simulink model "actuatorController"  (R2025b)
settings: Solver=FixedStepDiscrete  StartTime=0.0  StopTime=3  FixedStep=1e-3  RelTol=1e-3
undefined symbols (not defined in the file or in its folder): controller_mode, controller_modes, controllerGains, DiscIntNeverNeededParam
libraries: simulink x10, metux_library x4, eeGeneralControl x3, simulink_extras x2
settings Model: Creator=karadeli  LastModifiedBy=karadeli
settings OptimizationCC: GainParamInheritBuiltInType=on  UseFloatMulNetSlope=on  DefaultUnderspecifiedDataType=single  PassReuseOutputArgsAs=Individual arguments  ZeroExternalMemoryAtStartup=off  ZeroInternalMemoryAtStartup=off  NoFixptDivByZeroProtection=on  EfficientFloat2IntCast=on  LifeSpan=1  OptimizeBlockOrder=speed  DifferentSizesBufferReuse=on  EfficientTunableParamExpr=on
settings DebuggingCC: ParamSuppressDoubleToSinglePrecisionLossMsg=on  ParameterTunabilityLossMsg=none
settings HardwareCC: ProdBitPerPointer=32.0  ProdBitPerSizeT=32.0  ProdBitPerPtrDiffT=32.0  ProdLargestAtomicInteger=Long  ProdLargestAtomicFloat=Double  ProdWordSize=32.0  ProdLongLongMode=on  ProdHWDeviceType=ARM Compatible->ARM Cortex-M
settings SFSimCC: MATLABDynamicMemAlloc=off
settings RTWCC: SystemTargetFile=ert.tlc  GenCodeOnly=on  TemplateMakefile=ert_default_tmf  TargetLang=C++  Description=Embedded Coder
settings CodeAppCC: ForceParamTrailComments=on  IgnoreCustomStorageClasses=off  OperatorAnnotations=on  SimulinkDataObjDesc=on  SFDataObjDesc=on  CustomSymbolStrGlobalVar=rt$N$M  CustomSymbolStrType=$N$M  CustomSymbolStrFcn=$N$M$F  CustomSymbolStrMacro=$N$M  InsertBlockDesc=on
settings ERTTargetCC: InlinedParameterPlacement=Hierarchical  RootIOFormat=Structure reference  ERTCustomFileTemplate=example_file_process.tlc  ERTFilePackagingFormat=CompactWithDataFile  TargetLangStandard=C++11 (ISO)  GenerateSampleERTMain=on  IncludeMdlTerminateFcn=off  CombineSignalStateStructs=on  SupportAbsoluteTime=off  CodeInterfacePackaging=C++ class  SubcomponentCodeInterfacePackaging=C++ class  SupportNonFinite=off  SupportComplex=off  SupportNonInlinedSFcns=on

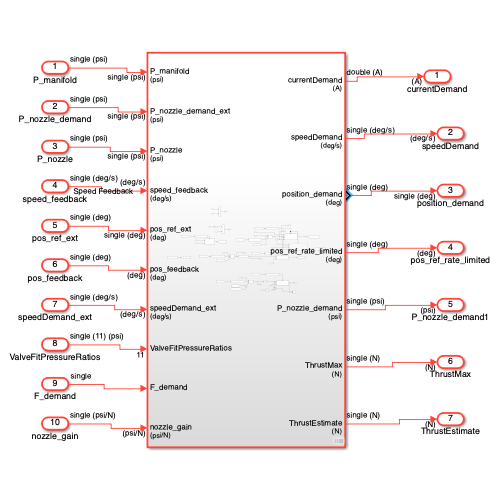
[thumbnail: Simulink's stored preview of the top-level diagram]
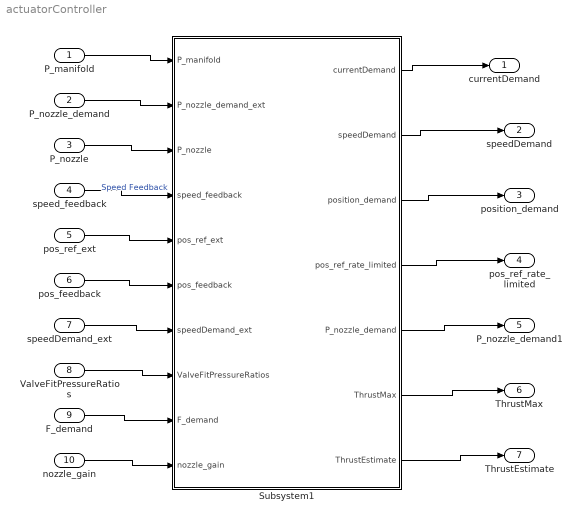
== system actuatorController ==
  P_manifold : Inport  OutDataTypeStr=single  Unit=psi  PortDimensions=1
  P_nozzle_demand : Inport  Port=2  OutDataTypeStr=single  Unit=psi  PortDimensions=1
  P_nozzle : Inport  Port=3  OutDataTypeStr=single  Unit=psi  PortDimensions=1
  speed_feedback : Inport  Port=4  Unit=deg/s  SampleTime=controllerGains.speed.Ts  Interpolate=off
  pos_ref_ext : Inport  Port=5  OutDataTypeStr=single  Unit=deg  SampleTime=controllerGains.position.Ts  Interpolate=off
  pos_feedback : Inport  Port=6  Unit=deg  SampleTime=controllerGains.position.Ts  Interpolate=off
  speedDemand_ext : Inport  Port=7  Unit=deg/s
  ValveFitPressureRatios : Inport  Port=8
  F_demand : Inport  Port=9
  nozzle_gain : Inport  Port=10  Unit=psi/N
  Subsystem1 : Subsystem
  currentDemand : Outport  Unit=A
  speedDemand : Outport  Port=2  Unit=deg/s
  position_demand : Outport  Port=3  OutDataTypeStr=single  Unit=deg
  pos_ref_rate_limited : Outport  Port=4  Unit=deg
  P_nozzle_demand1 : Outport  Port=5  Unit=psi
  ThrustMax : Outport  Port=6  Unit=N
  ThrustEstimate : Outport  Port=7  Unit=N
  wires:
  speed_feedback/1 -> Subsystem1/4(speed_feedback)  "Speed Feedback"
  pos_ref_ext/1 -> Subsystem1/5(pos_ref_ext)
  pos_feedback/1 -> Subsystem1/6(pos_feedback)
  P_manifold/1 -> Subsystem1/1(P_manifold)
  P_nozzle_demand/1 -> Subsystem1/2(P_nozzle_demand_ext)
  P_nozzle/1 -> Subsystem1/3(P_nozzle)
  speedDemand_ext/1 -> Subsystem1/7(speedDemand_ext)
  Subsystem1/3(position_demand) -> position_demand/1
  Subsystem1/4(pos_ref_rate_limited) -> pos_ref_rate_limited/1
  Subsystem1/1(currentDemand) -> currentDemand/1
  Subsystem1/2(speedDemand) -> speedDemand/1
  ValveFitPressureRatios/1 -> Subsystem1/8(ValveFitPressureRatios)
  F_demand/1 -> Subsystem1/9(F_demand)
  nozzle_gain/1 -> Subsystem1/10(nozzle_gain)
  Subsystem1/5(P_nozzle_demand) -> P_nozzle_demand1/1
  Subsystem1/6(ThrustMax) -> ThrustMax/1
  Subsystem1/7(ThrustEstimate) -> ThrustEstimate/1

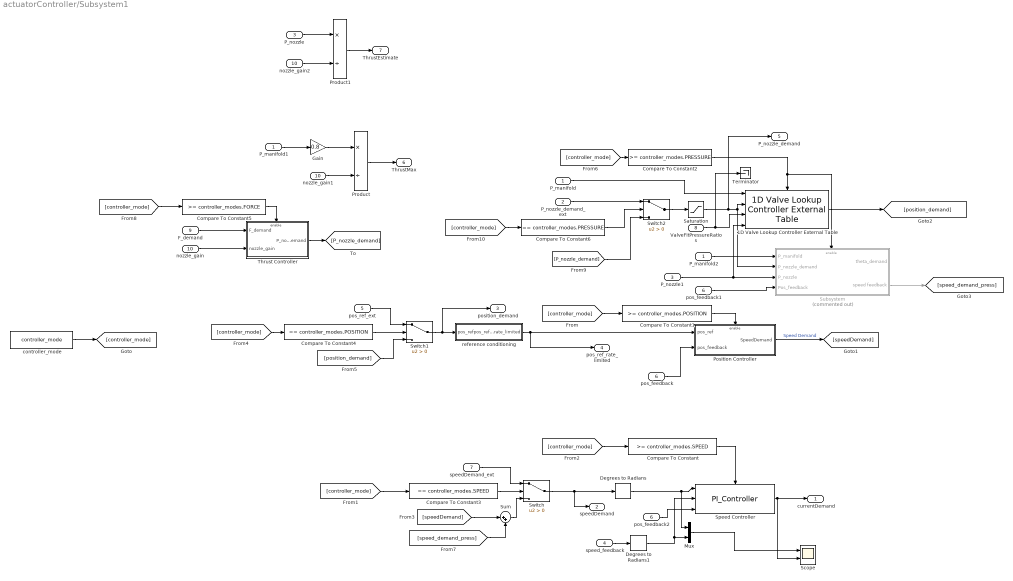
== system actuatorController/Subsystem1 ==
  P_manifold : Inport  OutDataTypeStr=single  Unit=psi  PortDimensions=1
  P_nozzle_demand_ext : Inport  Port=2  OutDataTypeStr=single  Unit=psi  PortDimensions=1
  P_nozzle : Inport  Port=3  OutDataTypeStr=single  Unit=psi  PortDimensions=1
  speed_feedback : Inport  Port=4  Unit=deg/s  SampleTime=controllerGains.speed.Ts  Interpolate=off
  pos_ref_ext : Inport  Port=5  OutDataTypeStr=single  Unit=deg  SampleTime=controllerGains.position.Ts  Interpolate=off
  pos_feedback : Inport  Port=6  Unit=deg  SampleTime=controllerGains.position.Ts  Interpolate=off
  speedDemand_ext : Inport  Port=7  Unit=deg/s
  ValveFitPressureRatios : Inport  Port=8
  F_demand : Inport  Port=9
  nozzle_gain : Inport  Port=10  Unit=psi/N
  1D Valve Lookup Controller External Table : metux_library/1D Valve Lookup Controller External Table  SystemSampleTime=-1  VariantActivationTime=update diagram  EmptyChoice=off  PassThrough=off  PassThroughVariantControl=(default)  EmptyChoiceVariantControl=(default)  AllowFlexibleInterface=on  Latency=0  AutoFrameSizeCalculation=off
  Compare To Constant : simulink/Logic and Bit Operations/Compare To Constant  relop=>=  const=controller_modes.SPEED  OutDataTypeStr=boolean
  Compare To Constant1 : simulink/Logic and Bit Operations/Compare To Constant  relop=>=  const=controller_modes.POSITION  OutDataTypeStr=boolean
  Compare To Constant2 : simulink/Logic and Bit Operations/Compare To Constant  relop=>=  const=controller_modes.PRESSURE  OutDataTypeStr=boolean
  Compare To Constant3 : simulink/Logic and Bit Operations/Compare To Constant  relop===  const=controller_modes.SPEED  OutDataTypeStr=boolean
  Compare To Constant4 : simulink/Logic and Bit Operations/Compare To Constant  relop===  const=controller_modes.POSITION  OutDataTypeStr=boolean
  Compare To Constant5 : simulink/Logic and Bit Operations/Compare To Constant  relop=>=  const=controller_modes.FORCE  OutDataTypeStr=boolean
  Compare To Constant6 : simulink/Logic and Bit Operations/Compare To Constant  relop===  const=controller_modes.PRESSURE  OutDataTypeStr=boolean
  Degrees to Radians : simulink_extras/Transformations/Degrees to Radians
  Degrees to Radians1 : simulink_extras/Transformations/Degrees to Radians
  Gain : Gain  Gain=0.8
  Mux : Mux  Inputs=2
  P_manifold1 : InportShadow  OutDataTypeStr=single  Unit=psi  PortDimensions=1
  P_manifold2 : InportShadow  OutDataTypeStr=single  Unit=psi  PortDimensions=1
  P_nozzle1 : InportShadow  Port=3  OutDataTypeStr=single  Unit=psi  PortDimensions=1
  Position Controller : Subsystem
  Product : Product  Inputs=*/
  Product1 : Product  Inputs=*/
  Saturation : Saturate  UpperLimit=1800  LowerLimit=0
  Scope : Scope  NumInputPorts=2
      settings: ActiveDisplayYMinimum=-3482.2818450927725  ActiveDisplayYMaximum=28164.697982788086
  Speed Controller : metux_library/PI_Controller  Kp=controllerGains.speed.Kp  Ki=controllerGains.speed.Ki  SatMax=controllerGains.speed.SatMax  SatMin=controllerGains.speed.SatMin  Ts=controllerGains.speed.Ts  RateLimiterMax=controllerGains.speed.RateLimiterMax  RateLimiterMin=controllerGains.speed.RateLimiterMin
  Subsystem : Subsystem  Commented=on
  Sum : Sum  Inputs=|++
  Switch : Switch  Criteria=u2 > Threshold  SaturateOnIntegerOverflow=off  InputSameDT=off
  Switch1 : Switch  Criteria=u2 > Threshold  SaturateOnIntegerOverflow=off  InputSameDT=off
  Switch2 : Switch  Criteria=u2 > Threshold  SaturateOnIntegerOverflow=off  InputSameDT=off
  Terminator : Terminator
  Thrust Controller : Subsystem
  controller_mode : Constant  Value=controller_mode  SampleTime=-1
  nozzle_gain1 : InportShadow  Port=10  Unit=psi/N
  nozzle_gain2 : InportShadow  Port=10  Unit=psi/N
  pos_feedback1 : InportShadow  Port=6  Unit=deg  SampleTime=controllerGains.position.Ts  Interpolate=off
  pos_feedback2 : InportShadow  Port=6  Unit=deg  SampleTime=controllerGains.position.Ts  Interpolate=off
  reference conditioning : Subsystem
  currentDemand : Outport  Unit=A
  speedDemand : Outport  Port=2  Unit=deg/s
  position_demand : Outport  Port=3  OutDataTypeStr=single  Unit=deg
  pos_ref_rate_limited : Outport  Port=4  Unit=deg
  P_nozzle_demand : Outport  Port=5  Unit=psi
  ThrustMax : Outport  Port=6  Unit=N
  ThrustEstimate : Outport  Port=7  Unit=N
  wires:
  P_nozzle_demand_ext/1 -> Switch2/1
  [controller_mode] -> Compare To Constant4/1
  controller_mode/1 -> [controller_mode]
  speedDemand_ext/1 -> Switch/1
  Mux/1 -> Scope/1
  Sum/1 -> Switch/3
  speed_feedback/1 -> Degrees to Radians1/1
  Position Controller/1(SpeedDemand) -> [speedDemand]  "Speed Demand"
  Degrees to Radians/1 -> Mux/1, Speed Controller/1
  Switch/1 -> speedDemand/1, Degrees to Radians/1
  Compare To Constant1/1 -> Position Controller/Enable
  [controller_mode] -> Compare To Constant2/1
  Compare To Constant/1 -> Speed Controller/Enable
  pos_feedback/1 -> Position Controller/2(pos_feedback)
  Compare To Constant2/1 -> Subsystem/Enable, 1D Valve Lookup Controller External Table/Enable
  Compare To Constant4/1 -> Switch1/2
  [position_demand] -> Switch1/3
  [controller_mode] -> Compare To Constant1/1
  Speed Controller/1 -> currentDemand/1, Scope/2
  [controller_mode] -> Compare To Constant/1
  pos_ref_ext/1 -> Switch1/1
  Switch1/1 -> position_demand/1, reference conditioning/1(pos_ref)
  Degrees to Radians1/1 -> Speed Controller/2, Mux/2
  [controller_mode] -> Compare To Constant3/1
  Compare To Constant3/1 -> Switch/2
  reference conditioning/1(pos_ref_rate_limited) -> pos_ref_rate_limited/1, Position Controller/1(pos_ref)
  [speedDemand] -> Sum/1
  [speed_demand_press] -> Sum/2
  P_manifold/1 -> 1D Valve Lookup Controller External Table/1
  [controller_mode] -> Compare To Constant5/1
  Compare To Constant5/1 -> Thrust Controller/Enable
  ValveFitPressureRatios/1 -> Terminator/1, 1D Valve Lookup Controller External Table/3
  F_demand/1 -> Thrust Controller/1(F_demand)
  nozzle_gain/1 -> Thrust Controller/2(nozzle_gain)
  Thrust Controller/1(P_nozzle_demand) -> [P_nozzle_demand]
  Switch2/1 -> Saturation/1
  Compare To Constant6/1 -> Switch2/2
  [controller_mode] -> Compare To Constant6/1
  [P_nozzle_demand] -> Switch2/3
  P_manifold1/1 -> Gain/1
  nozzle_gain1/1 -> Product/2
  Product/1 -> ThrustMax/1
  Gain/1 -> Product/1
  P_nozzle/1 -> Product1/1
  nozzle_gain2/1 -> Product1/2
  Product1/1 -> ThrustEstimate/1
  P_nozzle1/1 -> 1D Valve Lookup Controller External Table/4, Subsystem/3(P_nozzle)
  pos_feedback1/1 -> Subsystem/4(Pos_feedback)
  P_manifold2/1 -> Subsystem/1(P_manifold)
  Subsystem/2(speed feedback) -> [speed_demand_press]
  1D Valve Lookup Controller External Table/1 -> [position_demand]
  pos_feedback2/1 -> Speed Controller/3
  Saturation/1 -> P_nozzle_demand/1, Subsystem/2(P_nozzle_demand), 1D Valve Lookup Controller External Table/2

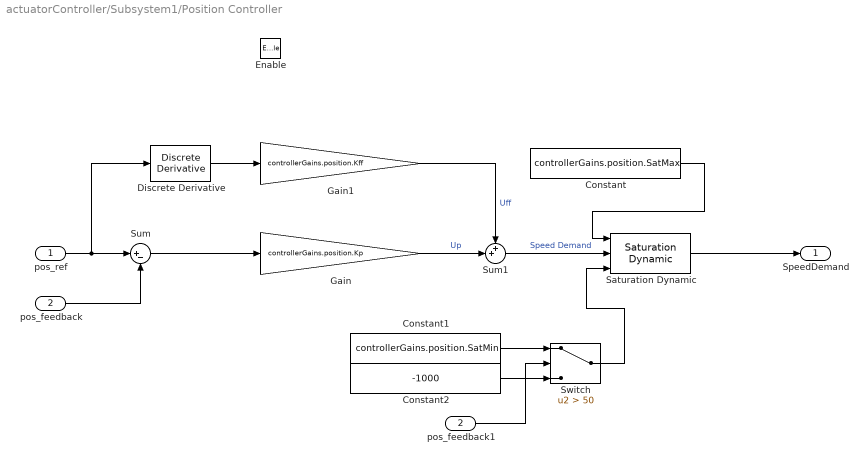
== system actuatorController/Subsystem1/Position Controller ==
  pos_ref : Inport  Unit=deg
  pos_feedback : Inport  Port=2  Unit=deg
  Enable : EnablePort  StatesWhenEnabling=reset
  Constant : Constant  Value=controllerGains.position.SatMax
  Constant1 : Constant  Value=controllerGains.position.SatMin
  Constant2 : Constant  Value=-1000  OutDataTypeStr=single
  Discrete Derivative : simulink/Discrete/Discrete Derivative  gainval=1.0  ICPrevScaledInput=0.0  OutMin=[]  OutMax=[]  OutDataType=fixdt(1, 16)  OutScaling=2^-10  DoSatur=off
  Gain : Gain  Gain=controllerGains.position.Kp
  Gain1 : Gain  Gain=controllerGains.position.Kff
  Saturation Dynamic : simulink/Discontinuities/Saturation Dynamic  OutMin=[]  OutMax=[]  OutDataTypeStr=Inherit: Same as second input  OutDataType=fixdt(1, 16)  OutScaling=2^-10  DoSatur=off
  Sum : Sum  Inputs=|+-
  Sum1 : Sum  Inputs=++|
  Switch : Switch  Criteria=u2 > Threshold  Threshold=50  SaturateOnIntegerOverflow=off  InputSameDT=off
  pos_feedback1 : InportShadow  Port=2  Unit=deg
  SpeedDemand : Outport  Unit=deg/s  OutputWhenDisabled=reset  InitialOutput=[0.0]
  wires:
  Saturation Dynamic/1 -> SpeedDemand/1
  pos_feedback/1 -> Sum/2
  Gain/1 -> Sum1/2  "Up"
  Sum/1 -> Gain/1
  pos_ref/1 -> Discrete Derivative/1, Sum/1
  Sum1/1 -> Saturation Dynamic/2  "Speed Demand"
  Discrete Derivative/1 -> Gain1/1
  Gain1/1 -> Sum1/1  "Uff"
  Constant/1 -> Saturation Dynamic/1
  Switch/1 -> Saturation Dynamic/3
  Constant1/1 -> Switch/1
  Constant2/1 -> Switch/3
  pos_feedback1/1 -> Switch/2

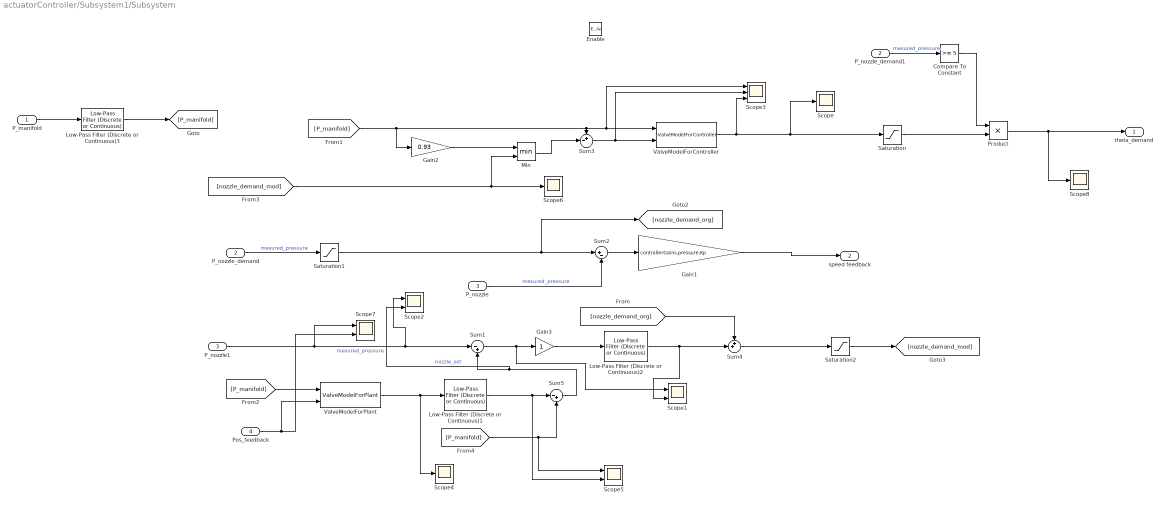
== system actuatorController/Subsystem1/Subsystem ==
  P_manifold : Inport
  P_nozzle_demand : Inport  Port=2
  P_nozzle : Inport  Port=3
  Pos_feedback : Inport  Port=4
  Enable : EnablePort  StatesWhenEnabling=reset
  Compare To Constant : simulink/Logic and Bit Operations/Compare To Constant  relop=>=  const=5  OutDataTypeStr=boolean
  Gain1 : Gain  Gain=controllerGains.pressure.Kp
  Gain2 : Gain  Gain=0.93
  Gain3 : Gain
  Low-Pass Filter (Discrete or Continuous)1 : eeGeneralControl/Low-Pass Filter (Discrete or Continuous)  K=1  T=0.001  B=inf  A=-inf  init_option=Inherited from block input  x0=0  Ts=-1
  Low-Pass Filter (Discrete or Continuous)2 : eeGeneralControl/Low-Pass Filter (Discrete or Continuous)  K=1  T=0.004  B=250  A=-250  init_option=Inherited from block input  x0=0  Ts=-1
  Low-Pass Filter (Discrete or Continuous)3 : eeGeneralControl/Low-Pass Filter (Discrete or Continuous)  K=single(1)  T=single(0.005)  B=inf  A=-inf  init_option=Inherited from block input  x0=0  Ts=-1
  Min : MinMax  Inputs=2
  P_nozzle1 : InportShadow  Port=3
  P_nozzle_demand1 : InportShadow  Port=2
  Product : Product
  Saturation : Saturate  UpperLimit=1080  LowerLimit=0
  Saturation1 : Saturate  UpperLimit=4000  LowerLimit=0
  Saturation2 : Saturate  UpperLimit=4000  LowerLimit=0
  Scope{,4,6,8} (4 alike) : Scope
      Scope settings: ActiveDisplayYMinimum=-15.395192146301266  ActiveDisplayYMaximum=138.55672931671143  DataLoggingVariableName=ScopeData2
      Scope4 settings: ActiveDisplayYMinimum=1007.1971893310547  ActiveDisplayYMaximum=2357.6605987548828  DataLoggingVariableName=ScopeData6
      Scope6 settings: ActiveDisplayYMinimum=-112.49999999999997  ActiveDisplayYMaximum=1012.5  DataLoggingVariableName=ScopeData8
      Scope8 settings: ActiveDisplayYMinimum=-18.167575836181637  ActiveDisplayYMaximum=163.50818252563477  DataLoggingVariableName=ScopeData10
  Scope{1..2,5,7} (4 alike) : Scope  NumInputPorts=2
      Scope1 settings: ActiveDisplayYMinimum=16.466037750244148  ActiveDisplayYMaximum=359.39812850952148  DataLoggingVariableName=ScopeData4
      Scope2 settings: ActiveDisplayYMinimum=-179.26073789596555  ActiveDisplayYMaximum=1025.8466792106628  DataLoggingVariableName=ScopeData5
      Scope5 settings: ActiveDisplayYMinimum=1218.2213745117188  ActiveDisplayYMaximum=2587.3870239257812  DataLoggingVariableName=ScopeData7
      Scope7 settings: ActiveDisplayYMinimum=-62.757351875305176  ActiveDisplayYMaximum=64.080883979797363  DataLoggingVariableName=ScopeData9
  Scope3 : Scope  NumInputPorts=3
      settings: ActiveDisplayYMinimum=-431.94372558593739  ActiveDisplayYMaximum=3887.4935302734375  DataLoggingVariableName=ScopeData3
  Sum1 : Sum  Inputs=|-+
  Sum2 : Sum  Inputs=|+-
  Sum3 : Sum  Inputs=+-|  OutDataTypeStr=single
  Sum4 : Sum  Inputs=++|
  Sum5 : Sum  Inputs=|-+
  ValveModelForController : metux_library/ValveModelForController  alpha=51.8534  C_max=0.9197
  ValveModelForPlant : metux_library/ValveModelForPlant  C_max=0.9197  alpha=51.8534
  theta_demand : Outport  OutputWhenDisabled=reset  InitialOutput=0
  speed feedback : Outport  Port=2
  wires:
  Sum1/1 -> Gain3/1, Scope1/1
  Sum3/1 -> Scope3/2, ValveModelForController/2
  Low-Pass Filter (Discrete or Continuous)1/1 -> Sum5/1, Scope5/2
  ValveModelForPlant/1 -> Low-Pass Filter (Discrete or Continuous)1/1, Scope4/1
  P_nozzle/1 -> Sum2/2  "mesured_pressure"
  P_nozzle_demand1/1 -> Compare To Constant/1  "mesured_pressure"
  P_manifold/1 -> Low-Pass Filter (Discrete or Continuous)3/1
  [P_manifold] -> Sum3/1, Scope3/1, ValveModelForController/1, Gain2/1
  Saturation/1 -> Product/2
  Compare To Constant/1 -> Product/1
  Pos_feedback/1 -> ValveModelForPlant/2, Scope7/2
  [P_manifold] -> ValveModelForPlant/1
  Gain3/1 -> Low-Pass Filter (Discrete or Continuous)2/1
  Saturation2/1 -> [nozzle_demand_mod]
  Min/1 -> Sum3/2
  Low-Pass Filter (Discrete or Continuous)3/1 -> [P_manifold]
  Low-Pass Filter (Discrete or Continuous)2/1 -> Sum4/2, Scope1/2
  P_nozzle1/1 -> Sum1/1, Scope2/1, Scope7/1  "mesured_pressure"
  Gain2/1 -> Min/1
  [nozzle_demand_mod] -> Scope6/1, Min/2
  Sum5/1 -> Sum1/2, Scope2/2  "nozzle_est"
  Saturation1/1 -> [nozzle_demand_org], Sum2/1
  [P_manifold] -> Sum5/2, Scope5/1
  ValveModelForController/1 -> Scope3/3, Saturation/1, Scope/1
  Product/1 -> theta_demand/1, Scope8/1
  Sum2/1 -> Gain1/1
  [nozzle_demand_org] -> Sum4/1
  P_nozzle_demand/1 -> Saturation1/1  "mesured_pressure"
  Sum4/1 -> Saturation2/1
  Gain1/1 -> speed feedback/1

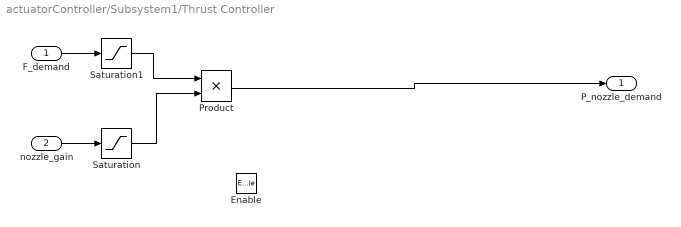
== system actuatorController/Subsystem1/Thrust Controller ==
  F_demand : Inport
  nozzle_gain : Inport  Port=2
  Enable : EnablePort
  Product : Product
  Saturation : Saturate  UpperLimit=inf  LowerLimit=0
  Saturation1 : Saturate  UpperLimit=inf  LowerLimit=0
  P_nozzle_demand : Outport
  wires:
  F_demand/1 -> Saturation1/1
  nozzle_gain/1 -> Saturation/1
  Saturation/1 -> Product/2
  Saturation1/1 -> Product/1
  Product/1 -> P_nozzle_demand/1

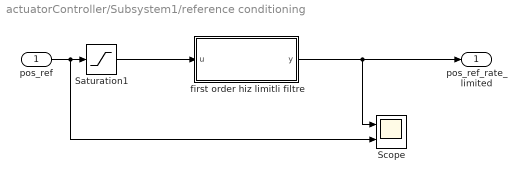
== system actuatorController/Subsystem1/reference conditioning ==
  pos_ref : Inport
  Saturation1 : Saturate  UpperLimit=360*4  LowerLimit=0
  Scope : Scope  NumInputPorts=2
      settings: ActiveDisplayYMinimum=115.37295030320635  ActiveDisplayYMaximum=137.10329135900082  DataLoggingVariableName=ScopeData11
  first order hiz limitli filtre : Subsystem
  pos_ref_rate_limited : Outport
  wires:
  pos_ref/1 -> Saturation1/1, Scope/2
  Saturation1/1 -> first order hiz limitli filtre/1(u)
  first order hiz limitli filtre/1(y) -> pos_ref_rate_limited/1, Scope/1

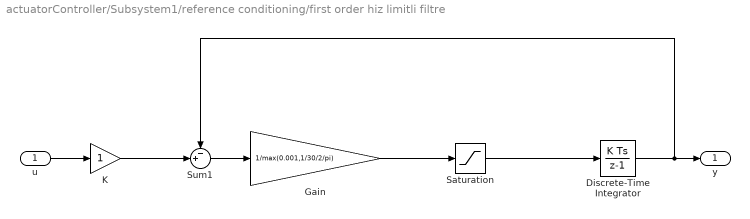
== system actuatorController/Subsystem1/reference conditioning/first order hiz limitli filtre ==
  u : Inport
  Discrete-Time Integrator : DiscreteIntegrator  SampleTime=-1  ICPrevOutput=DiscIntNeverNeededParam  ICPrevScaledInput=DiscIntNeverNeededParam
  Gain : Gain  Gain=1/max(0.001,1/30/2/pi)
  K : Gain
  Saturation : Saturate  UpperLimit=2400  LowerLimit=-2400
  Sum1 : Sum  Inputs=-+|
  y : Outport  VectorParamsAs1DForOutWhenUnconnected=off
  wires:
  K/1 -> Sum1/2
  Sum1/1 -> Gain/1
  Gain/1 -> Saturation/1
  Discrete-Time Integrator/1 -> Sum1/1, y/1
  u/1 -> K/1
  Saturation/1 -> Discrete-Time Integrator/1
